simulink model "lookup_table"  (R2022b)
settings: Solver=VariableStepAuto  StartTime=0.0  StopTime=inf  RelTol=1e-3
settings Model: Creator=user  LastModifiedBy=user

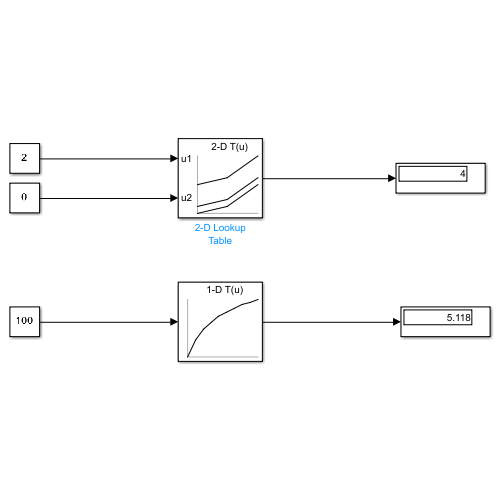
[thumbnail: Simulink's stored preview of the top-level diagram]
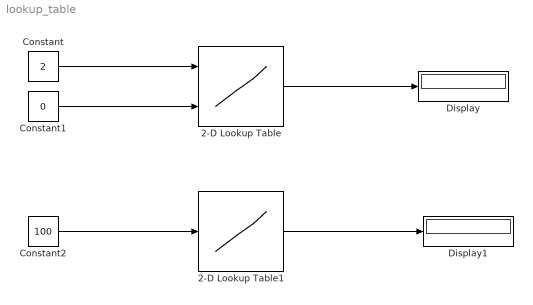
== system lookup_table ==
  2-D Lookup Table : Lookup_n-D  BreakpointsForDimension1=[0 1 2]  BreakpointsForDimension2=[0 : 2]  Table=[0 1 4; 1 2 5; 4 5 8]  InternalRulePriority=Speed  RndMeth=Simplest
      settings: InputPortMap=u0,u1
  2-D Lookup Table1 : Lookup_n-D  NumberOfTableDimensions=1  BreakpointsForDimension1=[1:10]  BreakpointsForDimension2=[0 : 2]  Table=log10([1:10])  InternalRulePriority=Speed  RndMeth=Simplest
  Constant : Constant  Value=2
  Constant1 : Constant  Value=0
  Constant2 : Constant  Value=100
  Display : Display
  Display1 : Display
  wires:
  Constant/1 -> 2-D Lookup Table/1
  Constant1/1 -> 2-D Lookup Table/2
  2-D Lookup Table/1 -> Display/1
  Constant2/1 -> 2-D Lookup Table1/1
  2-D Lookup Table1/1 -> Display1/1
